simulink model "lab5a"  (R2023b)
settings: Solver=VariableStepAuto  StartTime=0.0  StopTime=10.0  RelTol=1e-3
values from neighbouring files (symbols this model uses):
  Cf = [0.05, 0; 0, 0]    [lab5init.m]
  fd = [10, 0]    [lab5init.m]
  K = [1000, 0; 0, 0]    [lab5init.m]
  Kd = [5000, 0; 0, 5000]    [lab5init.m]
  Kp = [5000, 0; 0, 5000]    [lab5init.m]
  Md = [1000, 0; 0, 1000]    [lab5init.m]
  xe0 = [1.3, 0.7]    [lab5init.m]
  xr = [1.2, 0.7]    [lab5init.m]
undefined symbols (not defined in the file or in its folder): DiscIntNeverNeededParam
settings Model: Creator=rpl  LastModifiedBy=rpl

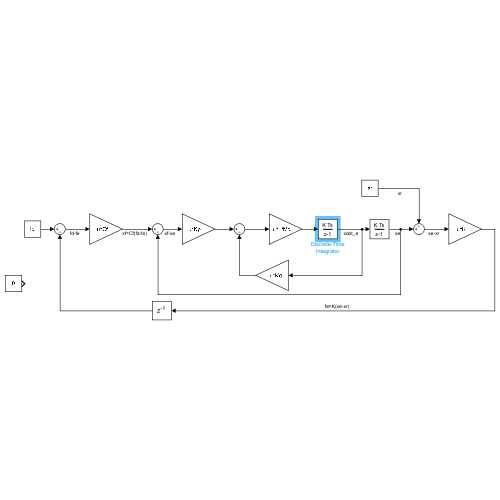
[thumbnail: Simulink's stored preview of the top-level diagram]
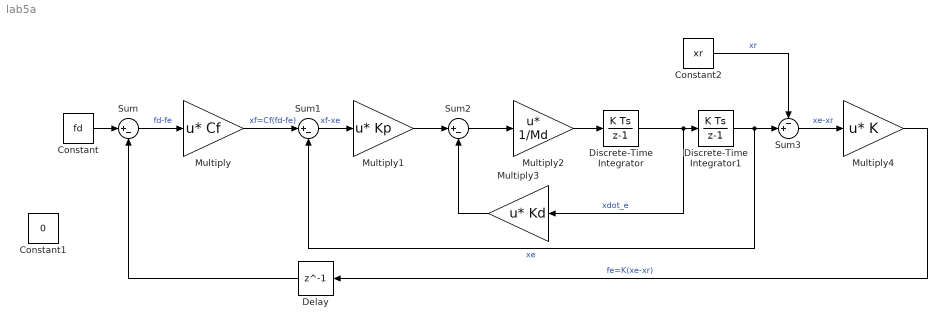
== system lab5a ==
  Constant : Constant  Value=fd  SampleTime=0.001
  Constant1 : Constant  Value=0
  Constant2 : Constant  Value=xr
  Delay : Delay  DelayLength=1  InitialCondition=xe0
  Discrete-Time Integrator : DiscreteIntegrator  SampleTime=-1  ICPrevOutput=DiscIntNeverNeededParam  ICPrevScaledInput=DiscIntNeverNeededParam
  Discrete-Time Integrator1 : DiscreteIntegrator  SampleTime=-1  ICPrevOutput=DiscIntNeverNeededParam  ICPrevScaledInput=DiscIntNeverNeededParam
  Multiply : Gain  Gain=Cf  Multiplication=Matrix(u*K)
  Multiply1 : Gain  Gain=Kp  Multiplication=Matrix(u*K)
  Multiply2 : Gain  Gain=1/Md  Multiplication=Matrix(u*K)
  Multiply3 : Gain  Gain=Kd  Multiplication=Matrix(u*K)
  Multiply4 : Gain  Gain=K  Multiplication=Matrix(u*K)
  Sum : Sum  Inputs=|+-
  Sum1 : Sum  Inputs=|+-
  Sum2 : Sum  Inputs=|+-
  Sum3 : Sum  Inputs=-+|
  wires:
  Constant/1 -> Sum/1
  Sum/1 -> Multiply/1  "fd-fe"
  Multiply/1 -> Sum1/1  "xf=Cf(fd-fe)"
  Sum1/1 -> Multiply1/1  "xf-xe"
  Multiply1/1 -> Sum2/1
  Sum2/1 -> Multiply2/1
  Multiply2/1 -> Discrete-Time Integrator/1
  Discrete-Time Integrator/1 -> Multiply3/1, Discrete-Time Integrator1/1  "xdot_e"
  Constant2/1 -> Sum3/1  "xr"
  Discrete-Time Integrator1/1 -> Sum1/2, Sum3/2  "xe"
  Sum3/1 -> Multiply4/1  "xe-xr"
  Multiply4/1 -> Delay/1  "fe=K(xe-xr)"
  Delay/1 -> Sum/2
  Multiply3/1 -> Sum2/2
